simulink model "MX28_simple"  (R2014b)
settings: Solver=ode45  StartTime=0.0  StopTime=1  RelTol=1e-6
undefined symbols (not defined in the file or in its folder): MX28_amplifier, MX28_dry_friction, MX28_inductor, MX28_inertia, MX28_init_position, MX28_init_speed, MX28_Kc, MX28_Kd, MX28_Ki, MX28_Kp, MX28_Kv, MX28_lub_friction, MX28_position_gain, MX28_reduction, MX28_resistor
libraries: simulink x1
settings Model: Creator=florent  LastModifiedBy=florent

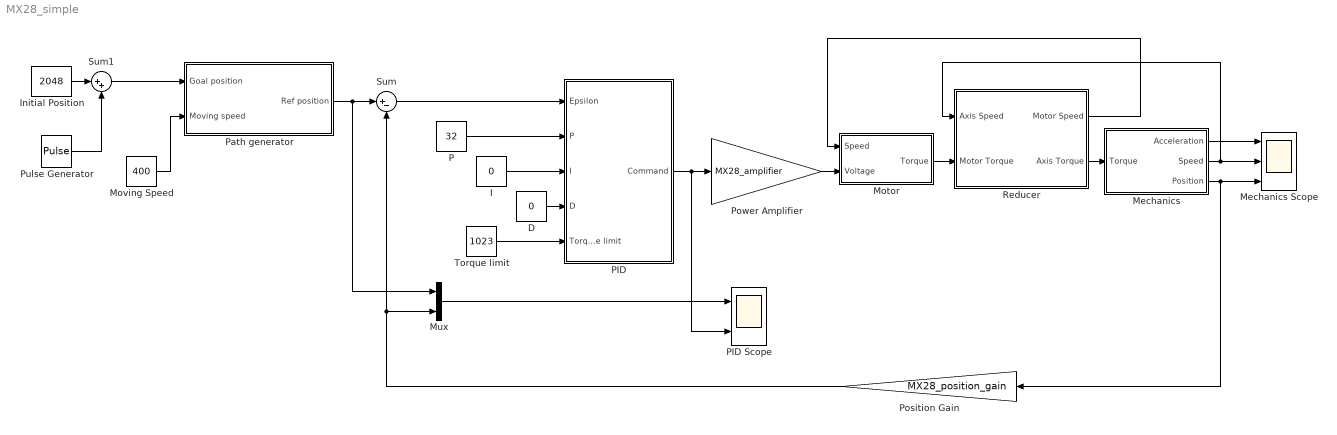
== system MX28_simple ==
  D : Constant  Value=0
  I : Constant  Value=0
  Initial Position : Constant  Value=2048  OutDataTypeStr=double
  Mechanics : Subsystem  TreatAsAtomicUnit=on
  Mechanics Scope : Scope  NumInputPorts=3
      settings: YMin=-5~-5~-5  YMax=5~5~5
  Motor : Subsystem
  Moving Speed : Constant  Value=400
  Mux : Mux  Inputs=2
  P : Constant  Value=32
  PID : Subsystem  TreatAsAtomicUnit=on
  PID Scope : Scope  NumInputPorts=2
      settings: YMin=0~-1000  YMax=2500~800
  Path generator : Subsystem  TreatAsAtomicUnit=on
  Position Gain : Gain  Gain=MX28_position_gain  OutMin=0  OutMax=4095  OutDataTypeStr=int16  RndMeth=Zero  SaturateOnIntegerOverflow=on
  Power Amplifier : Gain  Gain=MX28_amplifier  OutDataTypeStr=double
  Pulse Generator : DiscretePulseGenerator  PulseType=Time based  Amplitude=1024  Period=1  PulseWidth=50  PhaseDelay=0.1
  Reducer : Subsystem
  Sum : Sum  Inputs=|+-  AccumDataTypeStr=double  OutDataTypeStr=double  SaturateOnIntegerOverflow=on
  Sum1 : Sum  Inputs=|++  OutDataTypeStr=int16
  Torque limit : Constant  Value=1023
  wires:
  Motor/1(Torque) -> Reducer/2(Motor Torque)
  Power Amplifier/1 -> Motor/2(Voltage)
  Reducer/1(Motor Speed) -> Motor/1(Speed)
  Reducer/2(Axis Torque) -> Mechanics/1(Torque)
  Mechanics/2(Speed) -> Mechanics Scope/2, Reducer/1(Axis Speed)
  PID/1(Command) -> PID Scope/2, Power Amplifier/1
  P/1 -> PID/2(P)
  I/1 -> PID/3(I)
  D/1 -> PID/4(D)
  Sum/1 -> PID/1(Epsilon)
  Mechanics/3(Position) -> Position Gain/1, Mechanics Scope/3
  Position Gain/1 -> Mux/2, Sum/2
  Mechanics/1(Acceleration) -> Mechanics Scope/1
  Mux/1 -> PID Scope/1
  Initial Position/1 -> Sum1/1
  Pulse Generator/1 -> Sum1/2
  Torque limit/1 -> PID/5(Torque limit)
  Path generator/1(Ref position) -> Mux/1, Sum/1
  Sum1/1 -> Path generator/1(Goal position)
  Moving Speed/1 -> Path generator/2(Moving speed)

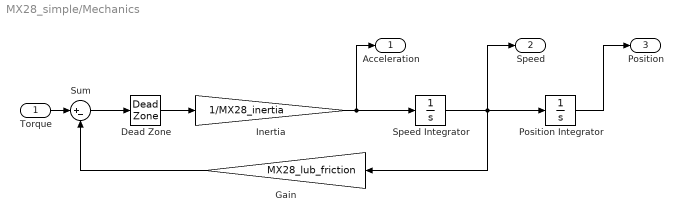
== system MX28_simple/Mechanics ==
  Torque : Inport
  Dead Zone : DeadZone  LowerValue=-MX28_dry_friction  UpperValue=MX28_dry_friction  SaturateOnIntegerOverflow=on
  Gain : Gain  Gain=MX28_lub_friction
  Inertia : Gain  Gain=1/MX28_inertia
  Position Integrator : Integrator  InitialCondition=MX28_init_position
  Speed Integrator : Integrator  InitialCondition=MX28_init_speed
  Sum : Sum  Inputs=|+-
  Acceleration : Outport
  Speed : Outport  Port=2
  Position : Outport  Port=3
  wires:
  Inertia/1 -> Acceleration/1, Speed Integrator/1
  Position Integrator/1 -> Position/1
  Torque/1 -> Sum/1
  Sum/1 -> Dead Zone/1
  Speed Integrator/1 -> Gain/1, Speed/1, Position Integrator/1
  Gain/1 -> Sum/2
  Dead Zone/1 -> Inertia/1

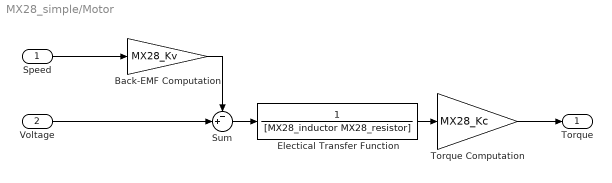
== system MX28_simple/Motor ==
  Speed : Inport
  Voltage : Inport  Port=2
  Back-EMF Computation : Gain  Gain=MX28_Kv
  Electical Transfer Function : TransferFcn  Denominator=[MX28_inductor MX28_resistor]
  Sum : Sum  Inputs=-+|
  Torque Computation : Gain  Gain=MX28_Kc
  Torque : Outport
  wires:
  Sum/1 -> Electical Transfer Function/1
  Voltage/1 -> Sum/2
  Back-EMF Computation/1 -> Sum/1
  Speed/1 -> Back-EMF Computation/1
  Torque Computation/1 -> Torque/1
  Electical Transfer Function/1 -> Torque Computation/1

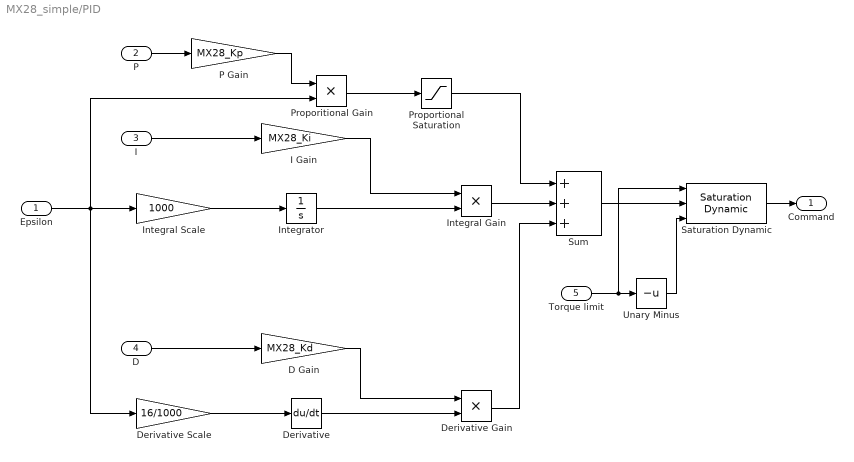
== system MX28_simple/PID ==
  Epsilon : Inport
  P : Inport  Port=2
  I : Inport  Port=3
  D : Inport  Port=4
  Torque limit : Inport  Port=5
  D Gain : Gain  Gain=MX28_Kd  OutDataTypeStr=double
  Derivative : Derivative
  Derivative Gain : Product
  Derivative Scale : Gain  Gain=16/1000
  I Gain : Gain  Gain=MX28_Ki  OutDataTypeStr=double
  Integral Gain : Product
  Integral Scale : Gain  Gain=1000
  Integrator : Integrator
  P Gain : Gain  Gain=MX28_Kp  OutDataTypeStr=double
  Proporitional Gain : Product
  Proportional Saturation : Saturate  UpperLimit=987  LowerLimit=-987
  Saturation Dynamic : simulink/Discontinuities/Saturation Dynamic  OutMin=[]  OutMax=[]  OutDataTypeStr=Inherit: Same as second input  OutDataType=fixdt(1, 16)  OutScaling=2^-10  DoSatur=off
  Sum : Sum  Inputs=+++  OutDataTypeStr=double  SaturateOnIntegerOverflow=on
  Unary Minus : UnaryMinus
  Command : Outport
  wires:
  Epsilon/1 -> Proporitional Gain/2, Integral Scale/1, Derivative Scale/1
  Sum/1 -> Saturation Dynamic/2
  Derivative Gain/1 -> Sum/3
  P/1 -> P Gain/1
  I/1 -> I Gain/1
  Integral Gain/1 -> Sum/2
  D/1 -> D Gain/1
  Derivative/1 -> Derivative Gain/2
  Proporitional Gain/1 -> Proportional Saturation/1
  Proportional Saturation/1 -> Sum/1
  Integral Scale/1 -> Integrator/1
  Derivative Scale/1 -> Derivative/1
  P Gain/1 -> Proporitional Gain/1
  I Gain/1 -> Integral Gain/1
  D Gain/1 -> Derivative Gain/1
  Integrator/1 -> Integral Gain/2
  Saturation Dynamic/1 -> Command/1
  Torque limit/1 -> Saturation Dynamic/1, Unary Minus/1
  Unary Minus/1 -> Saturation Dynamic/3

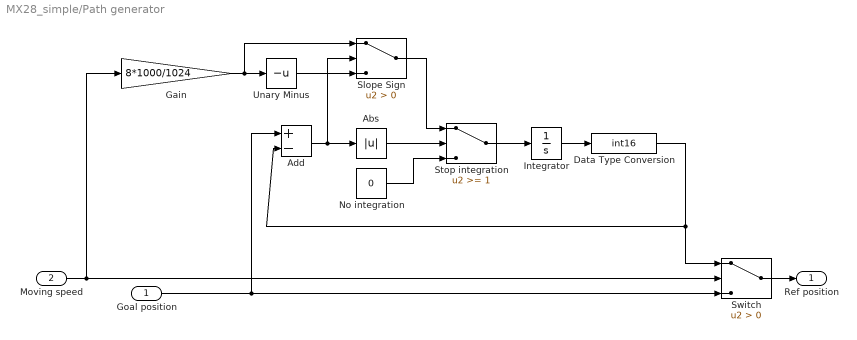
== system MX28_simple/Path generator ==
  Goal position : Inport
  Moving speed : Inport  Port=2
  Abs : Abs
  Add : Sum  Inputs=+-
  Data Type Conversion : DataTypeConversion  OutDataTypeStr=int16
  Gain : Gain  Gain=8*1000/1024
  Integrator : Integrator  InitialCondition=2048
  No integration : Constant  Value=0
  Slope Sign : Switch  Criteria=u2 > Threshold
  Stop integration : Switch  Threshold=1
  Switch : Switch  Criteria=u2 > Threshold
  Unary Minus : UnaryMinus
  Ref position : Outport
  wires:
  Moving speed/1 -> Gain/1, Switch/2
  Goal position/1 -> Switch/3, Add/1
  Switch/1 -> Ref position/1
  Integrator/1 -> Data Type Conversion/1
  Stop integration/1 -> Integrator/1
  No integration/1 -> Stop integration/3
  Abs/1 -> Stop integration/2
  Add/1 -> Slope Sign/2, Abs/1
  Slope Sign/1 -> Stop integration/1
  Unary Minus/1 -> Slope Sign/3
  Gain/1 -> Slope Sign/1, Unary Minus/1
  Data Type Conversion/1 -> Add/2, Switch/1

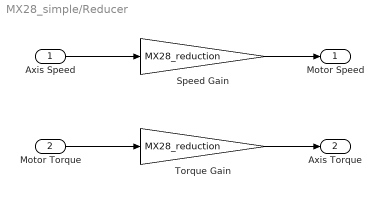
== system MX28_simple/Reducer ==
  Axis Speed : Inport
  Motor Torque : Inport  Port=2
  Speed Gain : Gain  Gain=MX28_reduction
  Torque Gain : Gain  Gain=MX28_reduction
  Motor Speed : Outport
  Axis Torque : Outport  Port=2
  wires:
  Torque Gain/1 -> Axis Torque/1
  Motor Torque/1 -> Torque Gain/1
  Axis Speed/1 -> Speed Gain/1
  Speed Gain/1 -> Motor Speed/1
